simulink library "ammclib_bam"  (Simulink 9.3)
settings: Solver=VariableStepAuto  StartTime=0.0  StopTime=10.0  RelTol=1e-3
undefined symbols (not defined in the file or in its folder): f16A1, f16A2, f16ADCMaxError, f16B0, f16B1, f16B2, f16C1, f16CC1, f16CC1sc, f16CC1sc_D, f16CC1sc_Q, f16CC2, f16CC2sc, f16CC2sc_D, f16CC2sc_Q, f16DerivGain, f16EGain, f16FiltCoef, f16HystOff, f16HystOn, f16IGain, f16IntegGain, f16IntegGainFW, f16IntegGainQ, f16Kd, f16Kq, f16Limit, f16LowerLimit, f16LowerLimit_D, f16LowerLimit_Q, f16LowerLimitFW, f16LowerLimitQ, f16ModIndex, f16OutValOff, f16OutValOn, f16PropGain, f16PropGainFW, f16PropGainQ, f16RampDown, f16RampUp, f16UGain, f16UpperLimit, f16UpperLimit_D, f16UpperLimit_Q, f16UpperLimitFW, f16UpperLimitQ, f16WIGain, f32A1, f32A2, f32ADCMaxError, f32B0, f32B1, f32B2, f32C1, f32CC1, f32CC1sc, f32CC1sc_D, f32CC1sc_Q, f32CC2, f32CC2sc ... (+114)
(part 9 of 21)

== system ammclib_bam/GDFLIB/F32 ==
  GDFLIB_FilterFIR_F32 : Subsystem  TreatAsAtomicUnit=on  mask(GDFLIB_FilterFIR_F32){u32Order=3, pCoefBuf=2^31*[0.25 0.25 0.25 0.25]}
      mask prompts: u32Order "u32Order (FIR filter order)"; pCoefBuf "pCoefBuf (FIR filter coefficients buffer. The array stores (u32Order + 1) filter coefficients.)"
      mask help: Finite impulse response filter in 32-bit fixed-point fractional implementation. Refer to the AMMCLIB User's Guide for further details.
      mask init: same as ammclib_bam/GDFLIB/F16/GDFLIB_FilterFIR_F16
      settings: RTWSystemCode=Inline
      mask Display: pos = get_param(gcb, 'Position');width = pos(3) - pos(1); height = pos(4) - pos(2);tX=width/2;tY=height - 8;color('black');text(tX,tY, 'GDFLIB_FilterFIR_F32', 'horizontalAlignment', 'center');
  GDFLIB_FilterIIR1_F32 : Subsystem  TreatAsAtomicUnit=on  mask(GDFLIB_FilterIIR1_F32){showStates=Hide (faster execution), f32B0=0, f32B1=0, f32A1=0}
      mask prompts: showStates "Show internal states"; f32B0 "f32B0 (B0 coefficient of the IIR1 filter in 32-bit fixed-point fractional format)"; f32B1 "f32B1 (B1 coefficient of the IIR1 filter in 32-bit fixed-point fractional format)"; f32A1 "f32A1 (A1 coefficient of the IIR1 filter in 32-bit fixed-point fractional format)"
      mask help: Direct form I first order IIR filter in 32-bit fixed-point fractional implementation. Refer to the AMMCLIB User's Guide for further details.
      mask init:
      | if ~evalin('base','exist(''tS8'',''var'')')
      |   if (2 ~= exist('SWLIBS_Typedefs.mat','file'))
      |       error('File SWLIBS_Typedefs.mat is not on the Matlab path. Please add the AMMCLIB "bam" folder in the Matlab Search Path.');
      |   else
      |       evalin('base', 'load(''SWLIBS_Typedefs.mat'')');
      |   end
      | end
      | if showStates == 1
      |     % hidden state variables
      |     if strcmp(get_param([gcb '/f32B0'], 'BlockType'), 'Inport')
      |         posblk = get_param(gcb, 'Position');
      | 
      |         pos = get_param(    [gcb, '/f32B0'], 'Position');
      |         orient = get_param( [gcb, '/f32B0'], 'Orientation');
      |         delete_block(       [gcb, '/f32B0']);
      |         add_block('built-in/Ground', [gcb, '/f32B0'], 'Position', pos, 'Orientation', orient);
      | 
      |         pos = get_param(    [gcb, '/f32B1'], 'Position');
      |         orient = get_param( [gcb, '/f32B1'], 'Orientation');
      |         delete_block(       [gcb, '/f32B1']);
      |         add_block('built-in/Ground', [gcb, '/f32B1'], 'Position', pos, 'Orientation', orient);
      | 
      |         pos = get_param(    [gcb, '/f32A1'], 'Position');
      |         orient = get_param( [gcb, '/f32A1'], 'Orientation');
      |         delete_block(       [gcb, '/f32A1']);
      |         add_block('built-in/Ground', [gcb, '/f32A1'], 'Position', pos, 'Orientation', orient);
      | 
      |         pos = get_param(    [gcb, '/f32FiltBufferX'], 'Position');
      |         orient = get_param( [gcb, '/f32FiltBufferX'], 'Orientation');
      |         delete_block(       [gcb, '/f32FiltBufferX']);
      |         add_block('built-in/Ground', [gcb, '/f32FiltBufferX'], 'Position', pos, 'Orientation', orient);
      | 
      |         pos = get_param(    [gcb, '/f32FiltBufferY'], 'Position');
      |         orient = get_param( [gcb, '/f32FiltBufferY'], 'Orientation');
      |         delete_block(       [gcb, '/f32FiltBufferY']);
      |         add_block('built-in/Ground', [gcb, '/f32FiltBufferY'], 'Position', pos, 'Orientation', orient);
      | 
      | 
      |         pos = get_param(    [gcb '/f32FiltBufferX_Out'], 'Position');
      |         orient = get_param( [gcb '/f32FiltBufferX_Out'], 'Orientation');
      |         delete_block(       [gcb '/f32FiltBufferX_Out']);
      |         add_block('built-in/Terminator', [gcb '/f32FiltBufferX_Out'], 'Position', pos, 'Orientation', orient);
      | 
      |         pos = get_param(    [gcb '/f32FiltBufferY_Out'], 'Position');
      |         orient = get_param( [gcb '/f32FiltBufferY_Out'], 'Orientation');
      |         delete_block(       [gcb '/f32FiltBufferY_Out']);
      |         add_block('built-in/Terminator', [gcb '/f32FiltBufferY_Out'], 'Position', pos, 'Orientation', orient);
      | 
      | 
      |         set_param([gcb '/f32In'], 'Port', '1');
      | 
      |         set_param([gcb '/f32Out'], 'Port', '1');
      | 
      |         set_param(gcb,'MaskEnables',{'on','on','on','on'});
      | 
      |         if (posblk(4) - posblk(2)) > 50
      |           height = 50;
      |           set_param(gcb,'Position',[posblk(1), posblk(2), posblk(3), posblk(2)+height])
      |         end
      |     end
      | else
      |     % shown state variables
      |     if strcmp(get_param([gcb '/f32B0'], 'BlockType'), 'Ground')
      |         posblk = get_param(gcb, 'Position');
      | 
      |         pos = get_param(    [gcb, '/f32B0'], 'Position');
      |         orient = get_param( [gcb, '/f32B0'], 'Orientation');
      |         delete_block(       [gcb, '/f32B0']);
      |         add_block('built-in/Inport', [gcb, '/f32B0'], 'Position', pos, 'Orientation', orient, 'OutDataTypeStr', 'int32');
      | 
      |         pos = get_param(    [gcb, '/f32B1'], 'Position');
      |         orient = get_param( [gcb, '/f32B1'], 'Orientation');
      |         delete_block(       [gcb, '/f32B1']);
      |         add_block('built-in/Inport', [gcb, '/f32B1'], 'Position', pos, 'Orientation', orient, 'OutDataTypeStr', 'int32');
      | 
      |         pos = get_param(    [gcb, '/f32A1'], 'Position');
      |         orient = get_param( [gcb, '/f32A1'], 'Orientation');
      |         delete_block(       [gcb, '/f32A1']);
      |         add_block('built-in/Inport', [gcb, '/f32A1'], 'Position', pos, 'Orientation', orient, 'OutDataTypeStr', 'int32');
      | 
      |         pos = get_param(    [gcb, '/f32FiltBufferX'], 'Position');
      |         orient = get_param( [gcb, '/f32FiltBufferX'], 'Orientation');
      |         delete_block(       [gcb, '/f32FiltBufferX']);
      |         add_block('built-in/Inport', [gcb, '/f32FiltBufferX'], 'Position', pos, 'Orientation', orient, 'OutDataTypeStr', 'int32');
      | 
      |         pos = get_param(    [gcb, '/f32FiltBufferY'], 'Position');
      |         orient = get_param( [gcb, '/f32FiltBufferY'], 'Orientation');
      |         delete_block(       [gcb, '/f32FiltBufferY']);
      |         add_block('built-in/Inport', [gcb, '/f32FiltBufferY'], 'Position', pos, 'Orientation', orient, 'OutDataTypeStr', 'int32');
      | 
      | 
      |         pos = get_param(    [gcb '/f32FiltBufferX_Out'], 'Position');
      |         orient = get_param( [gcb '/f32FiltBufferX_Out'], 'Orientation');
      |         delete_block(       [gcb '/f32FiltBufferX_Out']);
      |         add_block('built-in/Outport', [gcb '/f32FiltBufferX_Out'], 'Position', pos, 'Orientation', orient);
      | 
      |         pos = get_param(    [gcb '/f32FiltBufferY_Out'], 'Position');
      |         orient = get_param( [gcb '/f32FiltBufferY_Out'], 'Orientation');
      |         delete_block(       [gcb '/f32FiltBufferY_Out']);
      |         add_block('built-in/Outport', [gcb '/f32FiltBufferY_Out'], 'Position', pos, 'Orientation', orient);
      | 
      | 
      |         set_param([gcb '/f32In'], 'Port', '1');
      |         set_param([gcb '/f32B0'], 'Port', '2');
      |         set_param([gcb '/f32B1'], 'Port', '3');
      |         set_param([gcb '/f32A1'], 'Port', '4');
      |         set_param([gcb '/f32FiltBufferX'], 'Port', '5');
      |         set_param([gcb '/f32FiltBufferY'], 'Port', '6');
      | 
      |         set_param([gcb '/f32Out'], 'Port', '1');
      |         set_param([gcb '/f32FiltBufferX_Out'], 'Port', '2');
      |         set_param([gcb '/f32FiltBufferY_Out'], 'Port', '3');
      | 
      |         set_param(gcb,'MaskEnables',{'on','off','off','off'});
      | 
      |         if (posblk(4) - posblk(2)) < 175
      |           height = 175;
      |           set_param(gcb,'Position',[posblk(1), posblk(2), posblk(3), posblk(2)+height])
      |         end
      |     end
      | end
      settings: RTWSystemCode=Inline
      mask TypeOptions showStates: Hide (faster execution) | Show (allows debugging; connect feedback loops manually)
      mask Callback showStates:
      | maskStr = get_param(gcb,'showStates');
      | if strcmp(maskStr,'Hide (faster execution)'),
      |     set_param(gcb,'MaskEnables',{'on','on','on','on'});
      | else
      |     set_param(gcb,'MaskEnables',{'on','off','off','off'});
      | end
      mask Display:
      | color('black');
      | pos = get_param(gcb, 'Position');
      | width = pos(3) - pos(1);
      | height = pos(4) - pos(2);
      | tX=width/2;
      | tY=height - 8;
      | color('black');
      | text(tX,tY, 'GDFLIB_FilterIIR1_F32', 'horizontalAlignment', 'center');
      | if showStates == 2
      |   color('red');
      |   text(tX,tY - 20, ['debugging mode' char(13) char(10) '(limited performance)'], 'horizontalAlignment', 'center');
      | end
  GDFLIB_FilterIIR2_F32 : Subsystem  TreatAsAtomicUnit=on  mask(GDFLIB_FilterIIR2_F32){showStates=Hide (faster execution), f32B0=0, f32B1=0, f32B2=0, f32A1=0, f32A2=0}
      mask prompts: showStates "Show internal states"; f32B0 "f32B0 (B0 coefficient of the IIR2 filter in 32-bit fixed-point fractional format)"; f32B1 "f32B1 (B1 coefficient of the IIR2 filter in 32-bit fixed-point fractional format)"; f32B2 "f32B2 (B2 coefficient of the IIR2 filter in 32-bit fixed-point fractional format)"; f32A1 "f32A1 (A1 coefficient of the IIR2 filter in 32-bit fixed-point fractional format)"; f32A2 "f32A2 (A2 coefficient of the IIR2 filter in 32-bit fixed-point fractional format)"
      mask help: Direct form I second order IIR filter in 32-bit fixed-point fractional implementation. Refer to the AMMCLIB User's Guide for further details.
      mask init:
      | if ~evalin('base','exist(''tS8'',''var'')')
      |   if (2 ~= exist('SWLIBS_Typedefs.mat','file'))
      |       error('File SWLIBS_Typedefs.mat is not on the Matlab path. Please add the AMMCLIB "bam" folder in the Matlab Search Path.');
      |   else
      |       evalin('base', 'load(''SWLIBS_Typedefs.mat'')');
      |   end
      | end
      | if showStates == 1
      |     % hidden state variables
      |     if strcmp(get_param([gcb '/f32FiltBufferX1'], 'BlockType'), 'Inport')
      |         posblk = get_param(gcb, 'Position');
      | 
      |         pos = get_param(    [gcb, '/f32FiltBufferX1'], 'Position');
      |         orient = get_param( [gcb, '/f32FiltBufferX1'], 'Orientation');
      |         delete_block(       [gcb, '/f32FiltBufferX1']);
      |         add_block('built-in/Ground', [gcb, '/f32FiltBufferX1'], 'Position', pos, 'Orientation', orient);
      | 
      |         pos = get_param(    [gcb, '/f32FiltBufferX2'], 'Position');
      |         orient = get_param( [gcb, '/f32FiltBufferX2'], 'Orientation');
      |         delete_block(       [gcb, '/f32FiltBufferX2']);
      |         add_block('built-in/Ground', [gcb, '/f32FiltBufferX2'], 'Position', pos, 'Orientation', orient);
      | 
      |         pos = get_param(    [gcb, '/f32FiltBufferY1'], 'Position');
      |         orient = get_param( [gcb, '/f32FiltBufferY1'], 'Orientation');
      |         delete_block(       [gcb, '/f32FiltBufferY1']);
      |         add_block('built-in/Ground', [gcb, '/f32FiltBufferY1'], 'Position', pos, 'Orientation', orient);
      | 
      |         pos = get_param(    [gcb, '/f32FiltBufferY2'], 'Position');
      |         orient = get_param( [gcb, '/f32FiltBufferY2'], 'Orientation');
      |         delete_block(       [gcb, '/f32FiltBufferY2']);
      |         add_block('built-in/Ground', [gcb, '/f32FiltBufferY2'], 'Position', pos, 'Orientation', orient);
      | 
      |         pos = get_param(    [gcb, '/f32B0'], 'Position');
      |         orient = get_param( [gcb, '/f32B0'], 'Orientation');
      |         delete_block(       [gcb, '/f32B0']);
      |         add_block('built-in/Ground', [gcb, '/f32B0'], 'Position', pos, 'Orientation', orient);
      | 
      |         pos = get_param(    [gcb, '/f32B1'], 'Position');
      |         orient = get_param( [gcb, '/f32B1'], 'Orientation');
      |         delete_block(       [gcb, '/f32B1']);
      |         add_block('built-in/Ground', [gcb, '/f32B1'], 'Position', pos, 'Orientation', orient);
      | 
      |         pos = get_param(    [gcb, '/f32B2'], 'Position');
      |         orient = get_param( [gcb, '/f32B2'], 'Orientation');
      |         delete_block(       [gcb, '/f32B2']);
      |         add_block('built-in/Ground', [gcb, '/f32B2'], 'Position', pos, 'Orientation', orient);
      | 
      |         pos = get_param(    [gcb, '/f32A1'], 'Position');
      |         orient = get_param( [gcb, '/f32A1'], 'Orientation');
      |         delete_block(       [gcb, '/f32A1']);
      |         add_block('built-in/Ground', [gcb, '/f32A1'], 'Position', pos, 'Orientation', orient);
      | 
      |         pos = get_param(    [gcb, '/f32A2'], 'Position');
      |         orient = get_param( [gcb, '/f32A2'], 'Orientation');
      |         delete_block(       [gcb, '/f32A2']);
      |         add_block('built-in/Ground', [gcb, '/f32A2'], 'Position', pos, 'Orientation', orient);
      | 
      | 
      |         pos = get_param(    [gcb '/FilterBufferX1_Out'], 'Position');
      |         orient = get_param( [gcb '/FilterBufferX1_Out'], 'Orientation');
      |         delete_block(       [gcb '/FilterBufferX1_Out']);
      |         add_block('built-in/Terminator', [gcb '/FilterBufferX1_Out'], 'Position', pos, 'Orientation', orient);
      | 
      |         pos = get_param(    [gcb '/FilterBufferX2_Out'], 'Position');
      |         orient = get_param( [gcb '/FilterBufferX2_Out'], 'Orientation');
      |         delete_block(       [gcb '/FilterBufferX2_Out']);
      |         add_block('built-in/Terminator', [gcb '/FilterBufferX2_Out'], 'Position', pos, 'Orientation', orient);
      | 
      |         pos = get_param(    [gcb '/FilterBufferY1_Out'], 'Position');
      |         orient = get_param( [gcb '/FilterBufferY1_Out'], 'Orientation');
      |         delete_block(       [gcb '/FilterBufferY1_Out']);
      |         add_block('built-in/Terminator', [gcb '/FilterBufferY1_Out'], 'Position', pos, 'Orientation', orient);
      | 
      |         pos = get_param(    [gcb '/FilterBufferY2_Out'], 'Position');
      |         orient = get_param( [gcb '/FilterBufferY2_Out'], 'Orientation');
      |         delete_block(       [gcb '/FilterBufferY2_Out']);
      |         add_block('built-in/Terminator', [gcb '/FilterBufferY2_Out'], 'Position', pos, 'Orientation', orient);
      | 
      | 
      |         set_param([gcb '/f32In'], 'Port', '1');
      | 
      |         set_param([gcb '/f32Out'], 'Port', '1');
      | 
      |         set_param(gcb,'MaskEnables',{'on','on','on','on','on','on'});
      | 
      |         if (posblk(4) - posblk(2)) > 50
      |           height = 50;
      |           set_param(gcb,'Position',[posblk(1), posblk(2), posblk(3), posblk(2)+height])
      |         end
      |     end
      | else
      |     % shown state variables
      |     if strcmp(get_param([gcb '/f32FiltBufferX1'], 'BlockType'), 'Ground')
      |         posblk = get_param(gcb, 'Position');
      | 
      |         pos = get_param(    [gcb, '/f32FiltBufferX1'], 'Position');
      |         orient = get_param( [gcb, '/f32FiltBufferX1'], 'Orientation');
      |         delete_block(       [gcb, '/f32FiltBufferX1']);
      |         add_block('built-in/Inport', [gcb, '/f32FiltBufferX1'], 'Position', pos, 'Orientation', orient, 'OutDataTypeStr', 'int32');
      | 
      |         pos = get_param(    [gcb, '/f32FiltBufferX2'], 'Position');
      |         orient = get_param( [gcb, '/f32FiltBufferX2'], 'Orientation');
      |         delete_block(       [gcb, '/f32FiltBufferX2']);
      |         add_block('built-in/Inport', [gcb, '/f32FiltBufferX2'], 'Position', pos, 'Orientation', orient, 'OutDataTypeStr', 'int32');
      | 
      |         pos = get_param(    [gcb, '/f32FiltBufferY1'], 'Position');
      |         orient = get_param( [gcb, '/f32FiltBufferY1'], 'Orientation');
      |         delete_block(       [gcb, '/f32FiltBufferY1']);
      |         add_block('built-in/Inport', [gcb, '/f32FiltBufferY1'], 'Position', pos, 'Orientation', orient, 'OutDataTypeStr', 'int32');
      | 
      |         pos = get_param(    [gcb, '/f32FiltBufferY2'], 'Position');
      |         orient = get_param( [gcb, '/f32FiltBufferY2'], 'Orientation');
      |         delete_block(       [gcb, '/f32FiltBufferY2']);
      |         add_block('built-in/Inport', [gcb, '/f32FiltBufferY2'], 'Position', pos, 'Orientation', orient, 'OutDataTypeStr', 'int32');
      | 
      |         pos = get_param(    [gcb, '/f32B0'], 'Position');
      |         orient = get_param( [gcb, '/f32B0'], 'Orientation');
      |         delete_block(       [gcb, '/f32B0']);
      |         add_block('built-in/Inport', [gcb, '/f32B0'], 'Position', pos, 'Orientation', orient, 'OutDataTypeStr', 'int32');
      | 
      |         pos = get_param(    [gcb, '/f32B1'], 'Position');
      |         orient = get_param( [gcb, '/f32B1'], 'Orientation');
      |         delete_block(       [gcb, '/f32B1']);
      |         add_block('built-in/Inport', [gcb, '/f32B1'], 'Position', pos, 'Orientation', orient, 'OutDataTypeStr', 'int32');
      | 
      |         pos = get_param(    [gcb, '/f32B2'], 'Position');
      |         orient = get_param( [gcb, '/f32B2'], 'Orientation');
      |         delete_block(       [gcb, '/f32B2']);
      |         add_block('built-in/Inport', [gcb, '/f32B2'], 'Position', pos, 'Orientation', orient, 'OutDataTypeStr', 'int32');
      | 
      |         pos = get_param(    [gcb, '/f32A1'], 'Position');
      |         orient = get_param( [gcb, '/f32A1'], 'Orientation');
      |         delete_block(       [gcb, '/f32A1']);
      |         add_block('built-in/Inport', [gcb, '/f32A1'], 'Position', pos, 'Orientation', orient, 'OutDataTypeStr', 'int32');
      | 
      |         pos = get_param(    [gcb, '/f32A2'], 'Position');
      |         orient = get_param( [gcb, '/f32A2'], 'Orientation');
      |         delete_block(       [gcb, '/f32A2']);
      |         add_block('built-in/Inport', [gcb, '/f32A2'], 'Position', pos, 'Orientation', orient, 'OutDataTypeStr', 'int32');
      | 
      | 
      |         pos = get_param(    [gcb '/FilterBufferX1_Out'], 'Position');
      |         orient = get_param( [gcb '/FilterBufferX1_Out'], 'Orientation');
      |         delete_block(       [gcb '/FilterBufferX1_Out']);
      |         add_block('built-in/Outport', [gcb '/FilterBufferX1_Out'], 'Position', pos, 'Orientation', orient);
      | 
      |         pos = get_param(    [gcb '/FilterBufferX2_Out'], 'Position');
      |         orient = get_param( [gcb '/FilterBufferX2_Out'], 'Orientation');
      |         delete_block(       [gcb '/FilterBufferX2_Out']);
      |         add_block('built-in/Outport', [gcb '/FilterBufferX2_Out'], 'Position', pos, 'Orientation', orient);
      | 
      |         pos = get_param(    [gcb '/FilterBufferY1_Out'], 'Position');
      |         orient = get_param( [gcb '/FilterBufferY1_Out'], 'Orientation');
      |         delete_block(       [gcb '/FilterBufferY1_Out']);
      |         add_block('built-in/Outport', [gcb '/FilterBufferY1_Out'], 'Position', pos, 'Orientation', orient);
      | 
      |         pos = get_param(    [gcb '/FilterBufferY2_Out'], 'Position');
      |         orient = get_param( [gcb '/FilterBufferY2_Out'], 'Orientation');
      |         delete_block(       [gcb '/FilterBufferY2_Out']);
      |         add_block('built-in/Outport', [gcb '/FilterBufferY2_Out'], 'Position', pos, 'Orientation', orient);
      | 
      | 
      |         set_param([gcb '/f32In'], 'Port', '1');
      |         set_param([gcb '/f32FiltBufferX1'], 'Port', '2');
      |         set_param([gcb '/f32FiltBufferX2'], 'Port', '3');
      |         set_param([gcb '/f32FiltBufferY1'], 'Port', '4');
      |         set_param([gcb '/f32FiltBufferY2'], 'Port', '5');
      |         set_param([gcb '/f32B0'], 'Port', '6');
      |         set_param([gcb '/f32B1'], 'Port', '7');
      |         set_param([gcb '/f32B2'], 'Port', '8');
      |         set_param([gcb '/f32A1'], 'Port', '9');
      |         set_param([gcb '/f32A2'], 'Port', '10');
      | 
      |         set_param([gcb '/f32Out'], 'Port', '1');
      |         set_param([gcb '/FilterBufferX1_Out'], 'Port', '2');
      |         set_param([gcb '/FilterBufferX2_Out'], 'Port', '3');
      |         set_param([gcb '/FilterBufferY1_Out'], 'Port', '4');
      |         set_param([gcb '/FilterBufferY2_Out'], 'Port', '5');
      | 
      |         set_param(gcb,'MaskEnables',{'on','off','off','off','off','off'});
      | 
      |         if (posblk(4) - posblk(2)) < 275
      |           height = 275;
      |           set_param(gcb,'Position',[posblk(1), posblk(2), posblk(3), posblk(2)+height])
      |         end
      |     end
      | end
      settings: RTWSystemCode=Inline
      mask TypeOptions showStates: Hide (faster execution) | Show (allows debugging; connect feedback loops manually)
      mask Callback showStates:
      | maskStr = get_param(gcb,'showStates');
      | if strcmp(maskStr,'Hide (faster execution)'),
      |     set_param(gcb,'MaskEnables',{'on','on','on','on','on','on'});
      | else
      |     set_param(gcb,'MaskEnables',{'on','off','off','off','off','off'});
      | end
      mask Display:
      | color('black');
      | pos = get_param(gcb, 'Position');
      | width = pos(3) - pos(1);
      | height = pos(4) - pos(2);
      | tX=width/2;
      | tY=height - 8;
      | color('black');
      | text(tX,tY, 'GDFLIB_FilterIIR2_F32', 'horizontalAlignment', 'center');
      | if showStates == 2
      |   color('red');
      |   text(tX,tY - 20, ['debugging mode' char(13) char(10) '(limited performance)'], 'horizontalAlignment', 'center');
      | end
  GDFLIB_FilterMA_F32 : Subsystem  TreatAsAtomicUnit=on  mask(GDFLIB_FilterMA_F32){showStates=Hide (faster execution), resetStatesEnable=Pre-set according to the first set of inputs after reset, u16NSamples=0}
      mask prompts: showStates "Show internal states"; resetStatesEnable "Internal state after reset"; u16NSamples "u16NSamples (Recalculated smoothing factor in the range 0 to 31)"
      mask help: Exponential moving average filter in 32-bit fixed-point fractional implementation. This block supports re-initialization of the internal state during simulation. If the block is reset, the filter's output will be aligned with the input f32FilterMAOut_preset. Refer to the AMMCLIB User's Guide for further details.
      mask init:
      | if ~evalin('base','exist(''tS8'',''var'')')
      |   if (2 ~= exist('SWLIBS_Typedefs.mat','file'))
      |       error('File SWLIBS_Typedefs.mat is not on the Matlab path. Please add the AMMCLIB "bam" folder in the Matlab Search Path.');
      |   else
      |       evalin('base', 'load(''SWLIBS_Typedefs.mat'')');
      |   end
      | end
      | if showStates == 1
      |     % hidden state variables
      |     if strcmp(get_param([gcb '/u16NSamples'], 'BlockType'), 'Inport')
      |         posblk = get_param(gcb, 'Position');
      | 
      |         pos = get_param(    [gcb, '/u16NSamples'], 'Position');
      |         orient = get_param( [gcb, '/u16NSamples'], 'Orientation');
      |         delete_block(       [gcb, '/u16NSamples']);
      |         add_block('built-in/Ground', [gcb, '/u16NSamples'], 'Position', pos, 'Orientation', orient);
      | 
      |         pos = get_param(    [gcb, '/f32Acc'], 'Position');
      |         orient = get_param( [gcb, '/f32Acc'], 'Orientation');
      |         delete_block(       [gcb, '/f32Acc']);
      |         add_block('built-in/Ground', [gcb, '/f32Acc'], 'Position', pos, 'Orientation', orient);
      | 
      | 
      |         pos = get_param(    [gcb '/f32Acc_Out'], 'Position');
      |         orient = get_param( [gcb '/f32Acc_Out'], 'Orientation');
      |         delete_block(       [gcb '/f32Acc_Out']);
      |         add_block('built-in/Terminator', [gcb '/f32Acc_Out'], 'Position', pos, 'Orientation', orient);
      | 
      | 
      |         set_param([gcb '/f32In'], 'Port', '1');
      |         set_param([gcb '/f32FilterMAOut_preset'], 'Port', '2');
      | 
      |         set_param([gcb '/f32Out'], 'Port', '1');
      | 
      |         set_param(gcb,'MaskEnables',{'on','on','on'});
      | 
      |         if (posblk(4) - posblk(2)) > 75
      |           height = 75;
      |           set_param(gcb,'Position',[posblk(1), posblk(2), posblk(3), posblk(2)+height])
      |         end
      |     end
      | else
      |     % shown state variables
      |     if strcmp(get_param([gcb '/u16NSamples'], 'BlockType'), 'Ground')
      |         posblk = get_param(gcb, 'Position');
      | 
      |         pos = get_param(    [gcb, '/u16NSamples'], 'Position');
      |         orient = get_param( [gcb, '/u16NSamples'], 'Orientation');
      |         delete_block(       [gcb, '/u16NSamples']);
      |         add_block('built-in/Inport', [gcb, '/u16NSamples'], 'Position', pos, 'Orientation', orient, 'OutDataTypeStr', 'uint16');
      | 
      |         pos = get_param(    [gcb, '/f32Acc'], 'Position');
      |         orient = get_param( [gcb, '/f32Acc'], 'Orientation');
      |         delete_block(       [gcb, '/f32Acc']);
      |         add_block('built-in/Inport', [gcb, '/f32Acc'], 'Position', pos, 'Orientation', orient, 'OutDataTypeStr', 'int32');
      | 
      | 
      |         pos = get_param(    [gcb '/f32Acc_Out'], 'Position');
      |         orient = get_param( [gcb '/f32Acc_Out'], 'Orientation');
      |         delete_block(       [gcb '/f32Acc_Out']);
      |         add_block('built-in/Outport', [gcb '/f32Acc_Out'], 'Position', pos, 'Orientation', orient);
      | 
      | 
      |         set_param([gcb '/f32In'], 'Port', '1');
      |         set_param([gcb '/f32FilterMAOut_preset'], 'Port', '2');
      |         set_param([gcb '/u16NSamples'], 'Port', '3');
      |         set_param([gcb '/f32Acc'], 'Port', '4');
      | 
      |         set_param([gcb '/f32Out'], 'Port', '1');
      |         set_param([gcb '/f32Acc_Out'], 'Port', '2');
      | 
      |         set_param(gcb,'MaskEnables',{'on','on','off'});
      | 
      |         if (posblk(4) - posblk(2)) < 125
      |           height = 125;
      |           set_param(gcb,'Position',[posblk(1), posblk(2), posblk(3), posblk(2)+height])
      |         end
      |     end
      | end
      settings: RTWSystemCode=Inline
      mask TypeOptions showStates: Hide (faster execution) | Show (allows debugging; connect feedback loops manually)
      mask Callback showStates:
      | maskStr = get_param(gcb,'showStates');
      | if strcmp(maskStr,'Hide (faster execution)'),
      |     set_param(gcb,'MaskEnables',{'on','on','on'});
      | else
      |     set_param(gcb,'MaskEnables',{'on','on','off'});
      | end
      mask TypeOptions resetStatesEnable: Pre-set according to the first set of inputs after reset | Clear to zero
      mask Display:
      | color('black');
      | pos = get_param(gcb, 'Position');
      | width = pos(3) - pos(1);
      | height = pos(4) - pos(2);
      | tX=width/2;
      | tY=height - 25;
      | color('black');
      | text(tX,tY, 'GDFLIB_FilterMA_F32', 'horizontalAlignment', 'center');
      | if showStates == 2
      |   color('red');
      |   text(tX,tY - 20, ['debugging mode' char(13) char(10) '(limited performance)'], 'horizontalAlignment', 'center');
      | end
